simulink model "sys_2i2o"  (R2020a)
settings: Solver=VariableStepAuto  StartTime=0.0  StopTime=100  RelTol=1e-3
values from neighbouring files (symbols this model uses):
  Ts = 1/fs    (= 0.01)    [Model_2i2o.m]    (also in SystemIdentification.m = 0.001; exitationData.mat = 0.001; main_Simulink_Arduino_PIL_v05.m = 0.004; main_Simulink_Arduino_PIL_v05_v2.m)
undefined symbols (not defined in the file or in its folder): den11, den12, den21, den22, num11, num12, num21, num22
settings Model: Creator=Ricardo  LastModifiedBy=bezza
settings DataIOCC: ReturnWorkspaceOutputs=off
settings DebuggingCC: ArithmeticOperatorsInVariantConditions=warning
settings SFSimCC: SimUseLocalCustomCode=off  CustomCodeUndefinedFunction=UseInterfaceOnly
settings RTWCC: RTWUseLocalCustomCode=off
settings CodeAppCC: StateflowObjectComments=on

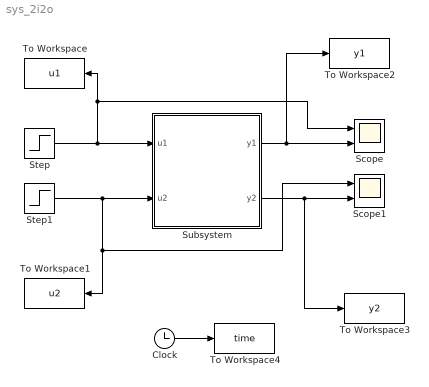
== system sys_2i2o ==
  Clock : Clock
  Scope : Scope  NumInputPorts=2
  Scope1 : Scope  NumInputPorts=2
  Step : Step  Time=20  Before=8.7402  After=8.8402  SampleTime=0
  Step1 : Step  Time=10  Before=9.256  After=9.356  SampleTime=0
  Subsystem : Subsystem
  To Workspace : ToWorkspace  VariableName=u1  SampleTime=Ts
  To Workspace1 : ToWorkspace  VariableName=u2  SampleTime=Ts
  To Workspace2 : ToWorkspace  VariableName=y1  SampleTime=Ts
  To Workspace3 : ToWorkspace  VariableName=y2  SampleTime=Ts
  To Workspace4 : ToWorkspace  VariableName=time  SampleTime=Ts
  wires:
  Step1/1 -> To Workspace1/1, Scope1/1, Subsystem/2(u2)
  Step/1 -> To Workspace/1, Scope/1, Subsystem/1(u1)
  Subsystem/1(y1) -> To Workspace2/1, Scope/2
  Subsystem/2(y2) -> To Workspace3/1, Scope1/2
  Clock/1 -> To Workspace4/1

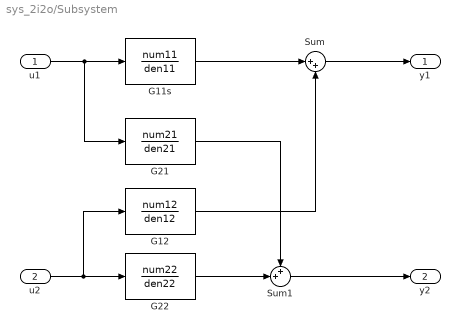
== system sys_2i2o/Subsystem ==
  u1 : Inport
  u2 : Inport  Port=2
  G11s : TransferFcn  Numerator=num11  Denominator=den11
  G12 : TransferFcn  Numerator=num12  Denominator=den12
  G21 : TransferFcn  Numerator=num21  Denominator=den21
  G22 : TransferFcn  Numerator=num22  Denominator=den22
  Sum : Sum  Inputs=|++
  Sum1 : Sum  Inputs=++|
  y1 : Outport
  y2 : Outport  Port=2
  wires:
  u2/1 -> G12/1, G22/1
  u1/1 -> G21/1, G11s/1
  G11s/1 -> Sum/1
  Sum/1 -> y1/1
  G22/1 -> Sum1/2
  Sum1/1 -> y2/1
  G21/1 -> Sum1/1
  G12/1 -> Sum/2
